simulink model "modelZSB_lib"  (Simulink 8.3)
settings: Solver=ode4  StartTime=0.0  StopTime=10  FixedStep=0.001  RelTol=1e-3
settings Model: Creator=Chan Hwaiwing  LastModifiedBy=shubo
settings DataIOCC: SignalLoggingSaveFormat=Dataset
settings DebuggingCC: UnderspecifiedInitializationDetection=Simplified  MergeDetectMultiDrivingBlocksExec=error  FrameProcessingCompatibilityMsg=error  StateNameClashWarn=none
settings GRTTargetCC: CombineOutputUpdateFcns=on  GRTInterface=off
settings ConfigComp: CovCompData="CovMetricSettings\t  dw"  CovFilter=CovHTMLOptions  CovHtmlReporting=on  CovSaveCumulativeToWorkspaceVar=on  CovSaveSingleToWorkspaceVar=on  CovModelRefExcluded="CovExternalEMLEnable\t  off"  CovSFcnEnable=off

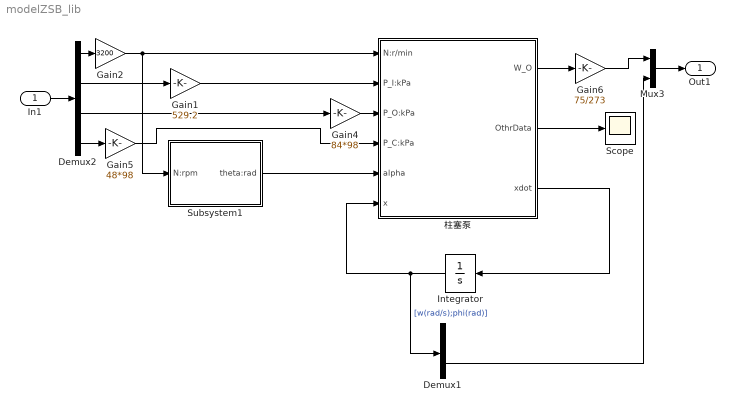
== system modelZSB_lib ==
  In1 : Inport
  Demux1 : Demux  Outputs=2
  Demux2 : Demux
  Gain1 : Gain  Gain=529.2
  Gain2 : Gain  Gain=3200
  Gain4 : Gain  Gain=84*98
  Gain5 : Gain  Gain=48*98
  Gain6 : Gain  Gain=75/273
  Integrator : Integrator  LimitOutput=on  UpperSaturationLimit=[inf 14.8/180*pi]  LowerSaturationLimit=[-inf 0/180*pi ]
  Mux3 : Mux  Inputs=2
  Scope : Scope
  Subsystem1 : Subsystem
  柱塞泵 : Subsystem  AncestorBlock=HMMtoolbox/泵类/ZSB  mask(柱塞泵){RHO=780, mode=平均模式, L_ZSBHX=15.02, D_ZSBZS=98.517, A_ZSBZS=23.8*23.8*pi/4, ETA_V=0.918, M_ZS=0.1006, Z_ZSBZS=7, BETA_ZSBZS=12/180*pi, A_ZSBTJ=[pi*(33.26^2-17^2)/4, pi*(33.26^2-19.8^2)/4], C_xp=[4.493 6.265 59.31 118.2], C_ea=[64.84 -11.88 15.36 59.23], k=31037.498, L_x0=205.554, J_ZSBXP=0.34*0.05, KD=7.65*0.5}
      mask prompts: RHO "RHO(标准状态下，油液密度kg/m^3)"; mode "计算模式"; L_ZSBHX "L_HX(等效滑靴厚度mm)"; D_ZSBZS "D_ZS(柱塞轴线在缸体的分布圆直径mm)"; A_ZSBZS "A_ZS(柱塞截面面积mm^2)"; ETA_V "ETA_V(容积效率)"; M_ZS "M_ZS(柱塞质量kg)"; Z_ZSBZS "Z_ZS(柱塞数量)"; BETA_ZSBZS "BETA_ZS(柱塞安装角rad)"; A_ZSBTJ "A_TJ(面积参数向量mm^2)"; C_xp "C_xp(3次多项式系数：斜盘角rad->活塞位移mm)"; C_ea "C_ea(3次多项式系数：斜盘角rad->等效力臂mm)"; k "k(弹簧弹性模量N/m)"; L_x0 "L_x0(弹簧自然长度mm)"; J_ZSBXP "J_XP(斜盘绕斜盘轴的转动惯量kg·m^2)"; KD "KD(斜盘转动阻力系数N·m·s/rad)"
      mask TypeOptions mode: 脉动模式 | 平均模式
      mask DialogControl DescTextVar Prompt: 填入相关参数
  Out1 : Outport
  wires:
  Integrator/1 -> 柱塞泵/6(x), Demux1/1  "[w(rad/s);phi(rad)]"
  Demux2/4 -> Gain5/1
  Demux2/3 -> Gain4/1
  Demux2/2 -> Gain1/1
  Subsystem1/1(theta:rad) -> 柱塞泵/5(alpha)
  In1/1 -> Demux2/1
  Demux2/1 -> Gain2/1
  柱塞泵/1(W_O) -> Gain6/1
  柱塞泵/3(xdot) -> Integrator/1
  柱塞泵/2(OthrData) -> Scope/1
  Gain2/1 -> 柱塞泵/1(N:r/min), Subsystem1/1(N:rpm)
  Gain1/1 -> 柱塞泵/2(P_I:kPa)
  Gain4/1 -> 柱塞泵/3(P_O:kPa)
  Gain5/1 -> 柱塞泵/4(P_C:kPa)
  Gain6/1 -> Mux3/1
  Mux3/1 -> Out1/1
  Demux1/2 -> Mux3/2

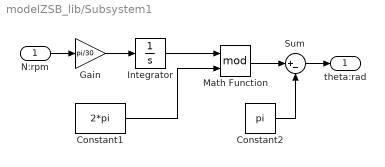
== system modelZSB_lib/Subsystem1 ==
  N:rpm : Inport
  Constant1 : Constant  Value=2*pi
  Constant2 : Constant  Value=pi
  Gain : Gain  Gain=pi/30
  Integrator : Integrator
  Math Function : Math  Operator=mod  SaturateOnIntegerOverflow=on
  Sum : Sum  Inputs=|+-
  theta:rad : Outport
  wires:
  Math Function/1 -> Sum/1
  N:rpm/1 -> Gain/1
  Constant1/1 -> Math Function/2
  Integrator/1 -> Math Function/1
  Gain/1 -> Integrator/1
  Sum/1 -> theta:rad/1
  Constant2/1 -> Sum/2

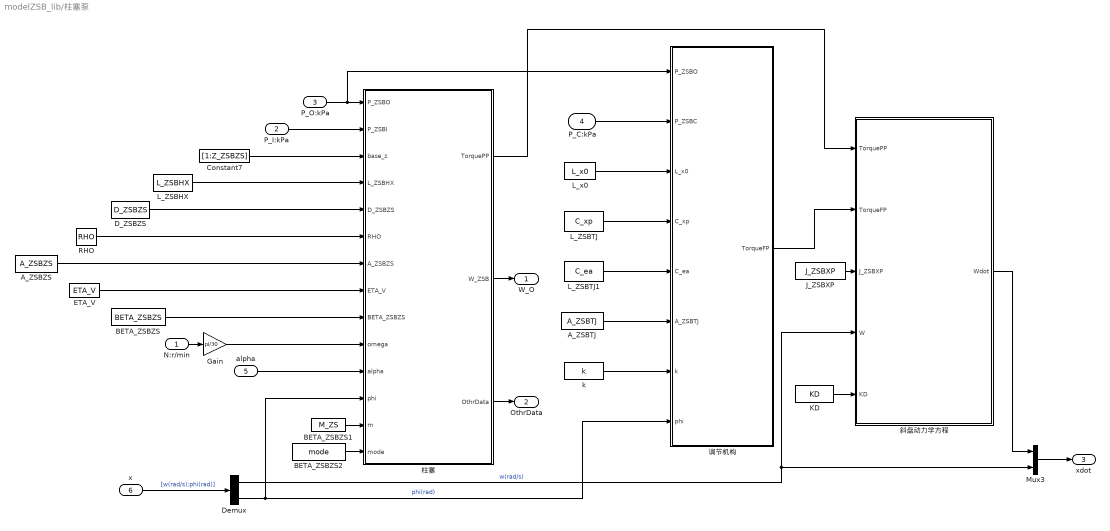
== system modelZSB_lib/柱塞泵 ==
  N:r/min : Inport
  P_I:kPa : Inport  Port=2
  P_O:kPa : Inport  Port=3
  P_C:kPa : Inport  Port=4
  alpha : Inport  Port=5
  x : Inport  Port=6
  A_ZSBTJ : Constant  Value=A_ZSBTJ
  A_ZSBZS : Constant  Value=A_ZSBZS
  BETA_ZSBZS : Constant  Value=BETA_ZSBZS
  BETA_ZSBZS1 : Constant  Value=M_ZS
  BETA_ZSBZS2 : Constant  Value=mode
  Constant7 : Constant  Value=[1:Z_ZSBZS]
  D_ZSBZS : Constant  Value=D_ZSBZS
  Demux : Demux  Outputs=2
  ETA_V : Constant  Value=ETA_V
  Gain : Gain  Gain=pi/30
  J_ZSBXP : Constant  Value=J_ZSBXP
  KD : Constant  Value=KD
  L_ZSBHX : Constant  Value=L_ZSBHX
  L_ZSBTJ : Constant  Value=C_xp
  L_ZSBTJ1 : Constant  Value=C_ea
  L_x0 : Constant  Value=L_x0
  Mux3 : Mux  Inputs=2
  RHO : Constant  Value=RHO
  k : Constant  Value=k
  斜盘动力学方程 : MATLAB Function  TreatAsAtomicUnit=on
  柱塞 : MATLAB Function  TreatAsAtomicUnit=on
  调节机构 : MATLAB Function  TreatAsAtomicUnit=on
  W_O : Outport
  OthrData : Outport  Port=2
  xdot : Outport  Port=3
  wires:
  x/1 -> Demux/1  "[w(rad/s);phi(rad)]"
  斜盘动力学方程/1(Wdot) -> Mux3/1
  Mux3/1 -> xdot/1
  柱塞/3(OthrData) -> OthrData/1
  alpha/1 -> 柱塞/11(alpha)
  J_ZSBXP/1 -> 斜盘动力学方程/3(J_ZSBXP)
  A_ZSBTJ/1 -> 调节机构/6(A_ZSBTJ)
  BETA_ZSBZS/1 -> 柱塞/9(BETA_ZSBZS)
  ETA_V/1 -> 柱塞/8(ETA_V)
  D_ZSBZS/1 -> 柱塞/5(D_ZSBZS)
  Demux/1 -> 斜盘动力学方程/4(W), Mux3/2  "w(rad/s)"
  柱塞/2(W_ZSB) -> W_O/1
  k/1 -> 调节机构/7(k)
  柱塞/1(TorquePP) -> 斜盘动力学方程/1(TorquePP)
  L_x0/1 -> 调节机构/3(L_x0)
  Gain/1 -> 柱塞/10(omega)
  P_O:kPa/1 -> 柱塞/1(P_ZSBO), 调节机构/1(P_ZSBO)
  L_ZSBTJ/1 -> 调节机构/4(C_xp)
  L_ZSBHX/1 -> 柱塞/4(L_ZSBHX)
  RHO/1 -> 柱塞/6(RHO)
  Constant7/1 -> 柱塞/3(base_z)
  A_ZSBZS/1 -> 柱塞/7(A_ZSBZS)
  N:r/min/1 -> Gain/1
  P_C:kPa/1 -> 调节机构/2(P_ZSBC)
  P_I:kPa/1 -> 柱塞/2(P_ZSBI)
  调节机构/1(TorqueFP) -> 斜盘动力学方程/2(TorqueFP)
  KD/1 -> 斜盘动力学方程/5(KD)
  BETA_ZSBZS1/1 -> 柱塞/13(m)
  BETA_ZSBZS2/1 -> 柱塞/14(mode)
  Demux/2 -> 调节机构/8(phi), 柱塞/12(phi)  "phi(rad)"
  L_ZSBTJ1/1 -> 调节机构/5(C_ea)

== matlab function 柱塞泵/斜盘动力学方程 ==
  data: TorquePP input double; Wdot output double; TorqueFP input double; J_ZSBXP input double; W input double; KD input double
function Wdot = DL(TorquePP,TorqueFP,J_ZSBXP,W, KD) 

    Torq_Net = TorquePP + TorqueFP - W * KD;
    Wdot =  Torq_Net / J_ZSBXP;
end

== matlab function 柱塞泵/柱塞 ==
  data: P_ZSBO input double; P_ZSBI input double; base_z input double; L_ZSBHX input double; D_ZSBZS input double; RHO input double; A_ZSBZS input double; ETA_V input double; BETA_ZSBZS input double; omega input double; alpha input double; TorquePP output double; W_ZSB output double; OthrData output double; phi input double; m input double; mode input double
function [ TorquePP, W_ZSB, OthrData ] = Plunger_Pump(P_ZSBO,  P_ZSBI,  base_z, L_ZSBHX, D_ZSBZS, RHO, A_ZSBZS, ETA_V,BETA_ZSBZS,omega,alpha,phi, m, mode )
r=D_ZSBZS/2;
z = length( base_z );
S_max = 2 * r * tan( phi );

if ( mode == 1 )
    
    alpha_tab =  alpha + base_z * 2 * pi / z;
    v_tab = -r * sin( alpha_tab ) * tan( phi ) * omega;
    l_tab = r * cos( alpha_tab ) / cos( phi ) + L_ZSBHX * tan( phi );

    p_tab = base_z;
    for i = 1 : z
        if ( alpha_tab( i ) >= pi )
            alpha_tab( i ) =  alpha_tab( i ) - 2 * pi;
        end
        if ( alpha_tab( i ) < 0 )
            p_tab( i ) = P_ZSBO;
        else
            p_tab( i ) = P_ZSBI;
            v_tab( i ) = 0;
        end
    end
    f1_tab = A_ZSBZS * p_tab / cos( phi );
    f2_tab = - r * m * tan( phi ) * omega * omega * cos( alpha_tab );
    f_tab = f1_tab + f2_tab;
    m_tab = l_tab .* f_tab * 1e-6;

    TorquePP = -sum( m_tab ); 
    q_tab = A_ZSBZS * ETA_V*cos(BETA_ZSBZS) * v_tab * RHO * 1e-9; 
    W_ZSB = sum( q_tab );
    OthrData = [ S_max, v_tab( z ), q_tab( z ), l_tab( z ), f_tab( z ), m_tab( z ) ];

else

    TorqueLG = 0.5*r*r*z*m*tan(phi)*omega*omega/cos(phi);
    TorqueYY = -0.5*z*L_ZSBHX*tan(phi)*A_ZSBZS*(P_ZSBO+P_ZSBI)/cos(phi);
    TorquePP = (TorqueYY + TorqueLG) * 1e-6;
    W_ZSB = RHO * ETA_V *cos(BETA_ZSBZS)* A_ZSBZS * S_max * z * omega * 0.5 / pi * 1e-9;
    OthrData = [ S_max, 0, 0, 0, 0, 0 ];
end

end

== matlab function 柱塞泵/调节机构 ==
  data: P_ZSBO input double; TorqueFP output double; P_ZSBC input double; L_x0 input double; C_xp input double; C_ea input double; A_ZSBTJ input double; k input double; phi input double
function TorqueFP= TJ( P_ZSBO, P_ZSBC, L_x0, C_xp, C_ea, A_ZSBTJ, k, phi)

% Displacement calculation
xp = C_xp(1) * phi ^3 + C_xp(2) * phi ^2 + C_xp(3) * phi +  C_xp(4);

% Force calculation
Pleft = P_ZSBO * 1e3;%kPa
Pright = Pleft-P_ZSBC * 1e3;%kPa
Fleft = Pleft * A_ZSBTJ(1) * 1e-6;%N
Fright = Pright * A_ZSBTJ(2) * 1e-6;%N
Fs = k * (L_x0 - xp) * 1e-3;
Fsui = Fs + Fright - Fleft;

% Equivalent Arm of Force & Torque
eqaf = C_ea(1) * phi ^3 + C_ea(2) * phi ^2 + C_ea(3) * phi +  C_ea(4);
TorqueFP = Fsui * eqaf * 1e-3;

end
